simulink model "problem5"  (R2020a)
settings: Solver=VariableStepAuto  StartTime=0.0  StopTime=10.0  RelTol=1e-3
model workspace (MAT data in the model file):
  C = 1e-05
  R = 10
undefined symbols (not defined in the file): q
settings Model: OrderedModelArguments=off  Creator=Jake  LastModifiedBy=Jake
settings DataIOCC: ExternalInput=[q]

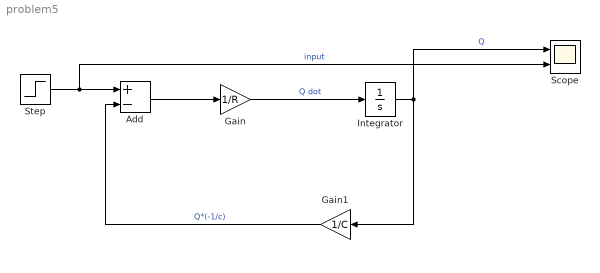
== system problem5 ==
  Add : Sum  Inputs=+-
  Gain : Gain  Gain=1/R
  Gain1 : Gain  Gain=1/C
  Integrator : Integrator  InitialCondition=q
  Scope : Scope  NumInputPorts=2
  Step : Step  SampleTime=0
  wires:
  Gain/1 -> Integrator/1  "Q dot"
  Gain1/1 -> Add/2  "Q*(-1/c)"
  Add/1 -> Gain/1
  Step/1 -> Scope/2, Add/1  "input"
  Integrator/1 -> Gain1/1, Scope/1  "Q"
